simulink model "rate_control_integrado_controlePD_r2018b"  (R2018b)
settings: Solver=FixedStepAuto  StartTime=0.0  StopTime=tsim  FixedStep=1/100  RelTol=1e-3
values from neighbouring files (symbols this model uses):
  Beff = 50    [Ex5.m]
  Jeff = 2.2    [Ex5.m]
  K = 17.7    [Ex5.m]
  Kd = (2*qsi*wn*Jeff - Beff)/K    (= -0.338983050847)    [Ex5.m]
  Kp = (wn^2*Jeff)/K    (= 12.4293785311)    [Ex5.m]
  L = [0.5;0.5;0.5]    [Ex5.m]
  N = 10    [Ex5.m]
  r = 1    [Ex5.m]
  SP_theta = ThetaA0    [Ex5.m]
  ThetaA0 = [10;20;30]    [Ex5.m]
  W_0 = [1 2 3]'    [Ex5.m]
  XdotC0 = [.2 -.3 -.2]'    [Ex5.m]
settings Model: Creator=Karoline  LastModifiedBy=Karoline
settings DataIOCC: ExternalInput=[L, ThetaA]
settings SFSimCC: SimUseLocalCustomCode=off
settings RTWCC: RTWUseLocalCustomCode=off
settings CodeAppCC: StateflowObjectComments=on

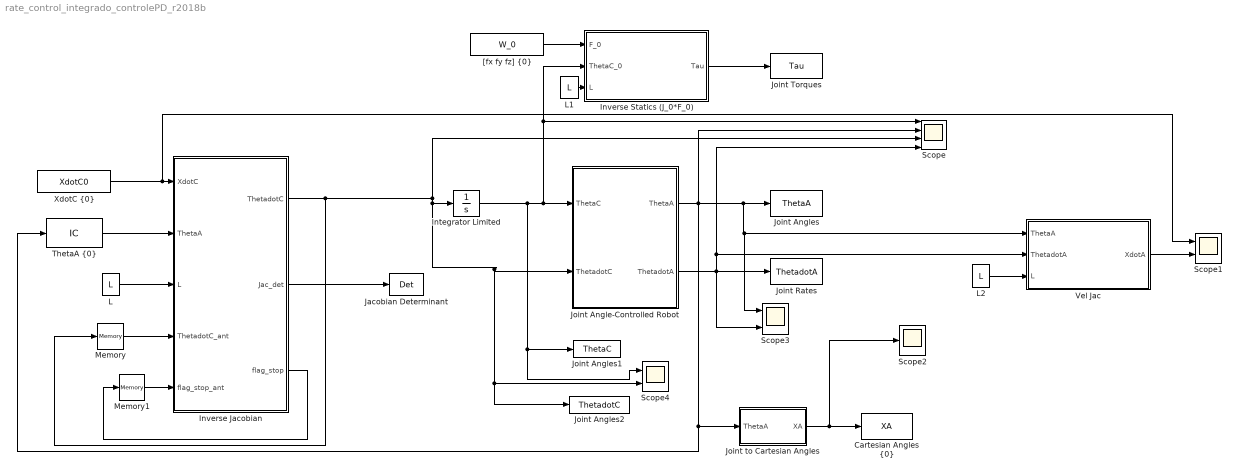
== system rate_control_integrado_controlePD_r2018b ==
  "Cartesian Angles {0}" : ToWorkspace  VariableName=XA  SampleTime=-1
      settings: Save2DSignal=2-D array (concatenate along first dimension)
  Integrator Limited : Integrator  InitialCondition=ThetaA0  LimitOutput=on  UpperSaturationLimit=[170, 170, 170]  LowerSaturationLimit=[-170, -170, -170]
  Inverse Jacobian : MATLAB Function  TreatAsAtomicUnit=on
  Inverse Statics (J_0*F_0) : MATLAB Function  TreatAsAtomicUnit=on
  Jacobian Determinant : ToWorkspace  VariableName=Det  SampleTime=-1
  Joint Angle-Controlled Robot : Subsystem
  Joint Angles : ToWorkspace  VariableName=ThetaA  SampleTime=-1
  Joint Angles1 : ToWorkspace  VariableName=ThetaC  SampleTime=-1
  Joint Angles2 : ToWorkspace  VariableName=ThetadotC  SampleTime=-1
  Joint Rates : ToWorkspace  VariableName=ThetadotA  SampleTime=-1
  Joint Torques : ToWorkspace  VariableName=Tau  SampleTime=-1
  Joint to Cartesian Angles : Subsystem
  L : Constant  Value=L
  L1 : Constant  Value=L
  L2 : Constant  Value=L
  Memory : Memory  InitialCondition=[0; 0; 0]
  Memory1 : Memory
  Scope : Scope  NumInputPorts=4
  Scope1 : Scope  NumInputPorts=2
  Scope2 : Scope
  Scope3 : Scope  NumInputPorts=2
  Scope4 : Scope  NumInputPorts=2
  "ThetaA {0}" : InitialCondition  Value=ThetaA0
  Vel Jac : MATLAB Function  TreatAsAtomicUnit=on
  "XdotC {0}" : Constant  Value=XdotC0
  "[fx fy fz] {0}" : Constant  Value=W_0
  wires:
  Inverse Jacobian/1(ThetadotC) -> Memory/1, Joint Angles2/1, Scope4/2, Joint Angle-Controlled Robot/2(ThetadotC), Integrator Limited/1, Scope/3
  Inverse Jacobian/2(Jac_det) -> Jacobian Determinant/1
  Integrator Limited/1 -> Joint Angles1/1, Scope4/1, Scope/1, Inverse Statics (J_0*F_0)/2(ThetaC_0), Joint Angle-Controlled Robot/1(ThetaC)
  Joint Angle-Controlled Robot/1(ThetaA) -> Scope/2, Scope3/1, Vel Jac/1(ThetaA), Joint Angles/1, "ThetaA {0}"/1, Joint to Cartesian Angles/1(ThetaA)
  Joint Angle-Controlled Robot/2(ThetadotA) -> Scope3/2, Scope/4, Vel Jac/2(ThetadotA), Joint Rates/1
  Inverse Statics (J_0*F_0)/1(Tau) -> Joint Torques/1
  Joint to Cartesian Angles/1(XA) -> Scope2/1, "Cartesian Angles {0}"/1
  "[fx fy fz] {0}"/1 -> Inverse Statics (J_0*F_0)/1(F_0)
  "ThetaA {0}"/1 -> Inverse Jacobian/2(ThetaA)
  L/1 -> Inverse Jacobian/3(L)
  L1/1 -> Inverse Statics (J_0*F_0)/3(L)
  L2/1 -> Vel Jac/3(L)
  Vel Jac/1(XdotA) -> Scope1/2
  Inverse Jacobian/3(flag_stop) -> Memory1/1
  "XdotC {0}"/1 -> Scope1/1, Inverse Jacobian/1(XdotC)
  Memory/1 -> Inverse Jacobian/4(ThetadotC_ant)
  Memory1/1 -> Inverse Jacobian/5(flag_stop_ant)

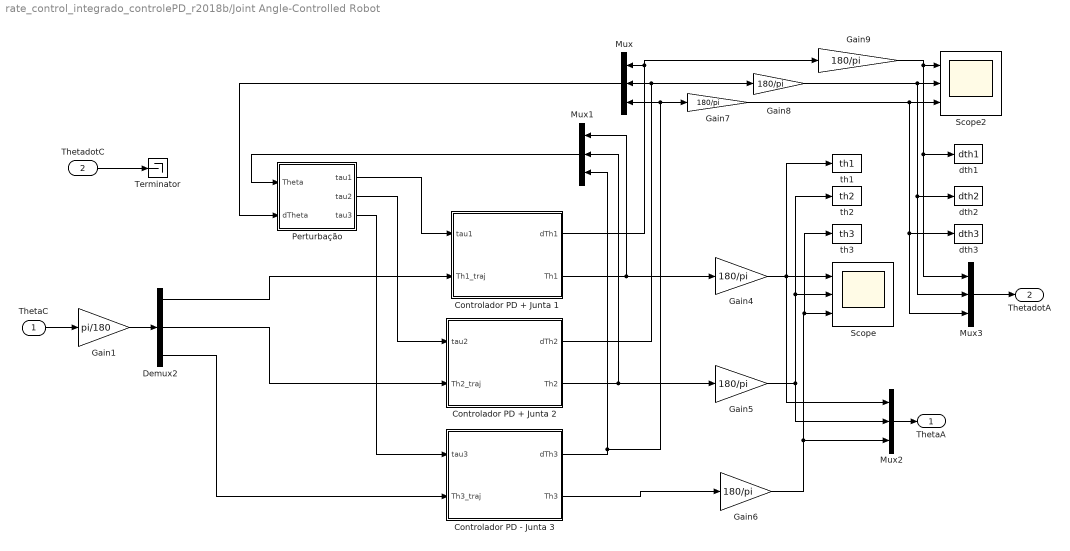
== system rate_control_integrado_controlePD_r2018b/Joint Angle-Controlled Robot ==
  ThetaC : Inport
  ThetadotC : Inport  Port=2
  Controlador PD + Junta 1 : Subsystem
  Controlador PD + Junta 2 : Subsystem
  Controlador PD - Junta 3 : Subsystem
  Demux2 : Demux  Outputs=3
  Gain1 : Gain  Gain=pi/180
  Gain{4..9} (6 alike) : Gain  Gain=180/pi
  Mux{,1..3} (4 alike) : Mux  Inputs=3
  Perturbação : Subsystem
  Scope : Scope  NumInputPorts=3
  Scope2 : Scope  NumInputPorts=3
  Terminator : Terminator
  dth1 : ToWorkspace  VariableName=dth1  SampleTime=-1
  dth2 : ToWorkspace  VariableName=dth2  SampleTime=-1
  dth3 : ToWorkspace  VariableName=dth3  SampleTime=-1
  th1 : ToWorkspace  VariableName=th1  SampleTime=-1
  th2 : ToWorkspace  VariableName=th2  SampleTime=-1
  th3 : ToWorkspace  VariableName=th3  SampleTime=-1
  ThetaA : Outport
  ThetadotA : Outport  Port=2
  wires:
  Gain8/1 -> Mux3/2, dth2/1, Scope2/2
  Gain9/1 -> Mux3/1, dth1/1, Scope2/1
  Controlador PD - Junta 3/1("dTh3 ") -> Mux1/3, Mux/3, Gain7/1
  Perturbação/3(tau3) -> Controlador PD - Junta 3/1(tau3)
  Gain7/1 -> Mux3/3, dth3/1, Scope2/3
  Gain5/1 -> th2/1, Scope/2, Mux2/2
  Controlador PD - Junta 3/2(Th3) -> Gain6/1
  Controlador PD + Junta 2/1("dTh2 ") -> Mux/2, Gain8/1
  Mux/1 -> Perturbação/2(dTheta)
  Controlador PD + Junta 2/2(Th2) -> Mux1/2, Gain5/1
  Gain4/1 -> th1/1, Mux2/1, Scope/1
  Controlador PD + Junta 1/1("dTh1 ") -> Mux/1, Gain9/1
  Perturbação/2(tau2) -> Controlador PD + Junta 2/1(tau2)
  Gain6/1 -> Mux2/3, th3/1, Scope/3
  Controlador PD + Junta 1/2(Th1) -> Mux1/1, Gain4/1
  Perturbação/1(tau1) -> Controlador PD + Junta 1/1(tau1)
  Mux1/1 -> Perturbação/1(Theta)
  ThetaC/1 -> Gain1/1
  Demux2/1 -> Controlador PD + Junta 1/2(Th1_traj)
  Demux2/2 -> Controlador PD + Junta 2/2(Th2_traj)
  Demux2/3 -> Controlador PD - Junta 3/2(Th3_traj)
  Mux2/1 -> ThetaA/1
  Mux3/1 -> ThetadotA/1
  Gain1/1 -> Demux2/1
  ThetadotC/1 -> Terminator/1

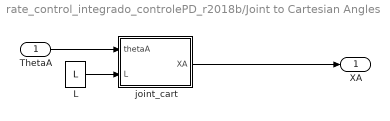
== system rate_control_integrado_controlePD_r2018b/Joint to Cartesian Angles ==
  ThetaA : Inport
  L : Constant  Value=L
  joint_cart : MATLAB Function  TreatAsAtomicUnit=on
  XA : Outport
  wires:
  ThetaA/1 -> joint_cart/1(thetaA)
  joint_cart/1(XA) -> XA/1
  L/1 -> joint_cart/2(L)

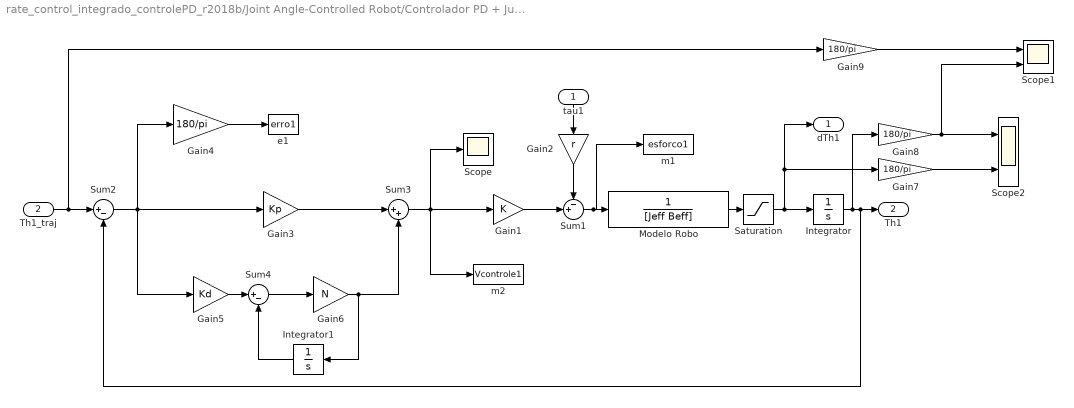
== system rate_control_integrado_controlePD_r2018b/Joint Angle-Controlled Robot/Controlador PD + Junta 1 ==
  tau1 : Inport
  Th1_traj : Inport  Port=2
  Gain1 : Gain  Gain=K
  Gain2 : Gain  Gain=r
  Gain3 : Gain  Gain=Kp
  Gain{4,7..9} (4 alike) : Gain  Gain=180/pi
  Gain5 : Gain  Gain=Kd
  Gain6 : Gain  Gain=N
  Integrator : Integrator  InitialCondition=SP_theta(1)*pi/180
  Integrator1 : Integrator
  Modelo Robo : TransferFcn  Denominator=[Jeff Beff]
  Saturation : Saturate  UpperLimit=10*pi/180  LowerLimit=-10*pi/180
  Scope : Scope
  Scope1 : Scope  NumInputPorts=2
  Scope2 : Scope  NumInputPorts=2
  Sum1 : Sum  Inputs=-+|
  Sum2 : Sum  Inputs=|+-
  Sum3 : Sum  Inputs=|++
  Sum4 : Sum  Inputs=|+-
  e1 : ToWorkspace  VariableName=erro1  SampleTime=-1
  m1 : ToWorkspace  VariableName=esforco1  SampleTime=-1
  m2 : ToWorkspace  VariableName=Vcontrole1  SampleTime=-1
  "dTh1 " : Outport
  Th1 : Outport  Port=2
  wires:
  tau1/1 -> Gain2/1
  Gain1/1 -> Sum1/2
  Sum1/1 -> m1/1, Modelo Robo/1
  Integrator/1 -> Gain8/1, Th1/1, Sum2/2
  Th1_traj/1 -> Gain9/1, Sum2/1
  Gain2/1 -> Sum1/1
  Sum2/1 -> Gain5/1, Gain3/1, Gain4/1
  Gain4/1 -> e1/1
  Gain3/1 -> Sum3/1
  Gain5/1 -> Sum4/1
  Sum4/1 -> Gain6/1
  Gain6/1 -> Sum3/2, Integrator1/1
  Integrator1/1 -> Sum4/2
  Sum3/1 -> m2/1, Scope/1, Gain1/1
  Modelo Robo/1 -> Saturation/1
  Saturation/1 -> "dTh1 "/1, Gain7/1, Integrator/1
  Gain8/1 -> Scope1/2, Scope2/1
  Gain7/1 -> Scope2/2
  Gain9/1 -> Scope1/1

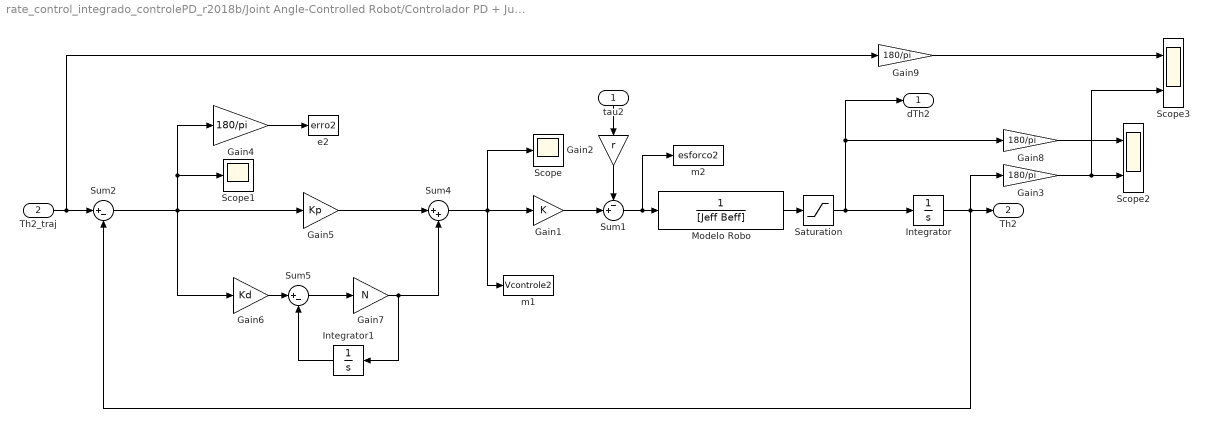
== system rate_control_integrado_controlePD_r2018b/Joint Angle-Controlled Robot/Controlador PD + Junta 2 ==
  tau2 : Inport
  Th2_traj : Inport  Port=2
  Gain1 : Gain  Gain=K
  Gain2 : Gain  Gain=r
  Gain{3..4,8..9} (4 alike) : Gain  Gain=180/pi
  Gain5 : Gain  Gain=Kp
  Gain6 : Gain  Gain=Kd
  Gain7 : Gain  Gain=N
  Integrator : Integrator  InitialCondition=SP_theta(2)*pi/180
  Integrator1 : Integrator
  "Modelo Robo " : TransferFcn  Denominator=[Jeff Beff]
  Saturation : Saturate  UpperLimit=10*pi/180  LowerLimit=-10*pi/180
  Scope : Scope
  Scope1 : Scope
  Scope2 : Scope  NumInputPorts=2
  Scope3 : Scope  NumInputPorts=2
  Sum1 : Sum  Inputs=-+|
  Sum2 : Sum  Inputs=|+-
  Sum4 : Sum  Inputs=|++
  Sum5 : Sum  Inputs=|+-
  e2 : ToWorkspace  VariableName=erro2  SampleTime=-1
  m1 : ToWorkspace  VariableName=Vcontrole2  SampleTime=-1
  m2 : ToWorkspace  VariableName=esforco2  SampleTime=-1
  "dTh2 " : Outport
  Th2 : Outport  Port=2
  wires:
  tau2/1 -> Gain2/1
  Gain1/1 -> Sum1/2
  Sum1/1 -> m2/1, "Modelo Robo "/1
  Integrator/1 -> Gain3/1, Th2/1, Sum2/2
  Gain2/1 -> Sum1/1
  Gain4/1 -> e2/1
  Gain5/1 -> Sum4/1
  Sum2/1 -> Gain4/1, Scope1/1, Gain6/1, Gain5/1
  Integrator1/1 -> Sum5/2
  Sum5/1 -> Gain7/1
  Gain6/1 -> Sum5/1
  Gain7/1 -> Sum4/2, Integrator1/1
  Sum4/1 -> m1/1, Scope/1, Gain1/1
  "Modelo Robo "/1 -> Saturation/1
  Saturation/1 -> Gain8/1, "dTh2 "/1, Integrator/1
  Gain3/1 -> Scope3/2, Scope2/2
  Gain8/1 -> Scope2/1
  Th2_traj/1 -> Gain9/1, Sum2/1
  Gain9/1 -> Scope3/1

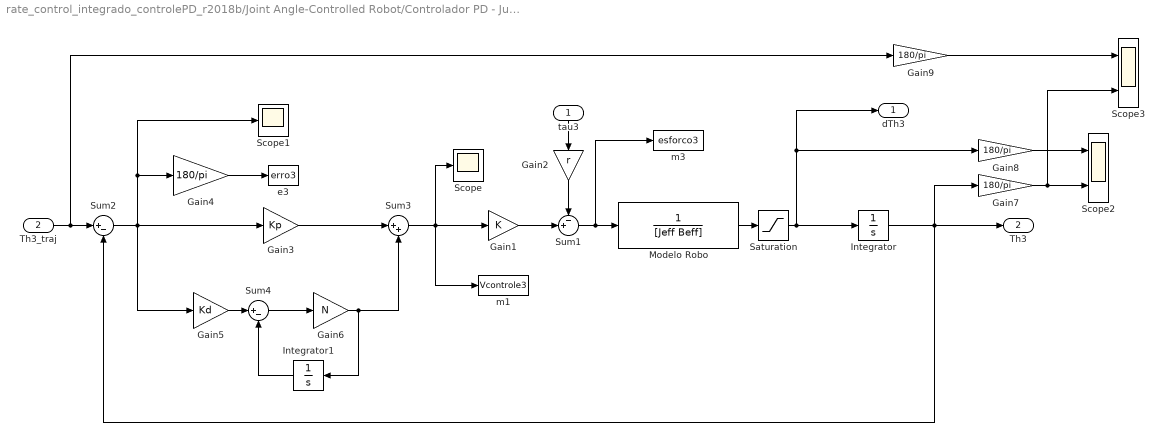
== system rate_control_integrado_controlePD_r2018b/Joint Angle-Controlled Robot/Controlador PD - Junta 3 ==
  tau3 : Inport
  Th3_traj : Inport  Port=2
  Gain1 : Gain  Gain=K
  Gain2 : Gain  Gain=r
  Gain3 : Gain  Gain=Kp
  Gain{4,7..9} (4 alike) : Gain  Gain=180/pi
  Gain5 : Gain  Gain=Kd
  Gain6 : Gain  Gain=N
  Integrator : Integrator  InitialCondition=SP_theta(3)*pi/180
  Integrator1 : Integrator
  Modelo Robo : TransferFcn  Denominator=[Jeff Beff]
  Saturation : Saturate  UpperLimit=10*pi/180  LowerLimit=-10*pi/180
  Scope : Scope
  Scope1 : Scope
  Scope2 : Scope  NumInputPorts=2
  Scope3 : Scope  NumInputPorts=2
  Sum1 : Sum  Inputs=-+|
  Sum2 : Sum  Inputs=|+-
  Sum3 : Sum  Inputs=|++
  Sum4 : Sum  Inputs=|+-
  e3 : ToWorkspace  VariableName=erro3  SampleTime=-1
  m1 : ToWorkspace  VariableName=Vcontrole3  SampleTime=-1
  m3 : ToWorkspace  VariableName=esforco3  SampleTime=-1
  "dTh3 " : Outport
  Th3 : Outport  Port=2
  wires:
  tau3/1 -> Gain2/1
  Gain1/1 -> Sum1/2
  Sum1/1 -> m3/1, Modelo Robo/1
  Integrator/1 -> Sum2/2, Gain7/1, Th3/1
  Th3_traj/1 -> Gain9/1, Sum2/1
  Gain2/1 -> Sum1/1
  Gain4/1 -> e3/1
  Gain3/1 -> Sum3/1
  Sum2/1 -> Gain4/1, Scope1/1, Gain5/1, Gain3/1
  Integrator1/1 -> Sum4/2
  Sum4/1 -> Gain6/1
  Gain5/1 -> Sum4/1
  Gain6/1 -> Sum3/2, Integrator1/1
  Sum3/1 -> m1/1, Scope/1, Gain1/1
  Modelo Robo/1 -> Saturation/1
  Saturation/1 -> Gain8/1, "dTh3 "/1, Integrator/1
  Gain7/1 -> Scope2/2, Scope3/2
  Gain8/1 -> Scope2/1
  Gain9/1 -> Scope3/1

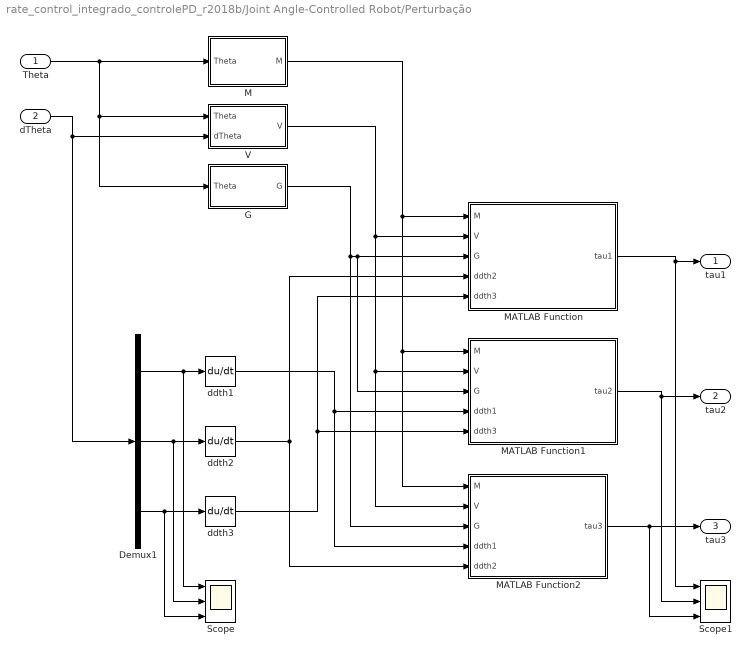
== system rate_control_integrado_controlePD_r2018b/Joint Angle-Controlled Robot/Perturbação ==
  Theta : Inport
  dTheta : Inport  Port=2
  Demux1 : Demux  Outputs=3
  G : Subsystem
  M : Subsystem
  MATLAB Function : MATLAB Function  TreatAsAtomicUnit=on
  MATLAB Function1 : MATLAB Function  TreatAsAtomicUnit=on
  MATLAB Function2 : MATLAB Function  TreatAsAtomicUnit=on
  Scope : Scope  NumInputPorts=3
  Scope1 : Scope  NumInputPorts=3
  V : Subsystem
  ddth1 : Derivative
  ddth2 : Derivative
  ddth3 : Derivative
  tau1 : Outport
  tau2 : Outport  Port=2
  tau3 : Outport  Port=3
  wires:
  dTheta/1 -> Demux1/1, V/2(dTheta)
  G/1(G) -> MATLAB Function2/3(G), MATLAB Function1/3(G), MATLAB Function/3(G)
  V/1(V) -> MATLAB Function/2(V), MATLAB Function1/2(V), MATLAB Function2/2(V)
  M/1(M) -> MATLAB Function2/1(M), MATLAB Function1/1(M), MATLAB Function/1(M)
  Theta/1 -> M/1(Theta), G/1(Theta), V/1(Theta)
  Demux1/1 -> Scope/1, ddth1/1
  Demux1/2 -> Scope/2, ddth2/1
  Demux1/3 -> Scope/3, ddth3/1
  ddth1/1 -> MATLAB Function2/4(ddth1), MATLAB Function1/4(ddth1)
  ddth3/1 -> MATLAB Function/5(ddth3), MATLAB Function1/5(ddth3)
  ddth2/1 -> MATLAB Function/4(ddth2), MATLAB Function2/5(ddth2)
  MATLAB Function/1(tau1) -> Scope1/1, tau1/1
  MATLAB Function1/1(tau2) -> tau2/1, Scope1/2
  MATLAB Function2/1(tau3) -> tau3/1, Scope1/3

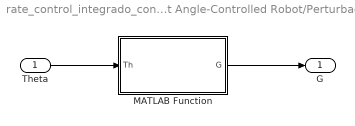
== system rate_control_integrado_controlePD_r2018b/Joint Angle-Controlled Robot/Perturbação/G ==
  Theta : Inport
  MATLAB Function : MATLAB Function  TreatAsAtomicUnit=on
  G : Outport
  wires:
  Theta/1 -> MATLAB Function/1(Th)
  MATLAB Function/1(G) -> G/1

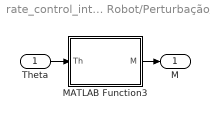
== system rate_control_integrado_controlePD_r2018b/Joint Angle-Controlled Robot/Perturbação/M ==
  Theta : Inport
  MATLAB Function3 : MATLAB Function  TreatAsAtomicUnit=on
  M : Outport
  wires:
  Theta/1 -> MATLAB Function3/1(Th)
  MATLAB Function3/1(M) -> M/1

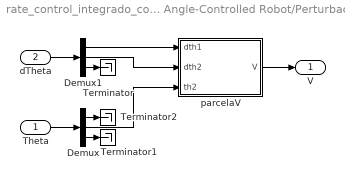
== system rate_control_integrado_controlePD_r2018b/Joint Angle-Controlled Robot/Perturbação/V ==
  Theta : Inport
  dTheta : Inport  Port=2
  Demux : Demux  Outputs=3
  Demux1 : Demux  Outputs=3
  Terminator : Terminator
  Terminator1 : Terminator
  Terminator2 : Terminator
  parcelaV : MATLAB Function  TreatAsAtomicUnit=on
  V : Outport
  wires:
  Theta/1 -> Demux/1
  dTheta/1 -> Demux1/1
  Demux1/1 -> parcelaV/1(dth1)
  Demux1/2 -> parcelaV/2(dth2)
  Demux/2 -> parcelaV/3(th2)
  parcelaV/1(V) -> V/1
  Demux1/3 -> Terminator/1
  Demux/1 -> Terminator2/1
  Demux/3 -> Terminator1/1

== matlab function rate_control_integrado_controlePD_r2018b/Inverse Jacobian ==
  data: XdotC input; ThetadotC output; ThetaA input; Jac_det output; L input; flag_stop output; ThetadotC_ant input; flag_stop_ant input
function [ThetadotC,Jac_det,flag_stop] = invjac(XdotC,ThetaA,L,ThetadotC_ant, flag_stop_ant)

vel_lim = 10; % º/seg

if (abs(ThetadotC_ant(1))>=vel_lim || abs(ThetadotC_ant(2))>=vel_lim || abs(ThetadotC_ant(3))>=vel_lim) || flag_stop_ant == 1
    ThetadotC = [0; 0; 0];
    flag_stop = 1;
    Jac_det = 0; %Jac_det_ant;
else
    [J] = jacobianRRR(ThetaA,L);
    Jac_det = det(J);
%     Jinv = inv(J);
    ThetadotC = J\XdotC;  
    
    flag_stop = 0;
end


end

== matlab function rate_control_integrado_controlePD_r2018b/Inverse Statics (J_0*F_0) ==
  data: F_0 input; Tau output; ThetaC_0 input; L input
function Tau = jacob_calcul(F_0,ThetaC_0,L)


J_0 = jacobianRRR(ThetaC_0,L); % jacobiano

Tau = J_0'*F_0;

== matlab function rate_control_integrado_controlePD_r2018b/Joint to Cartesian Angles/joint_cart ==
  data: thetaA input; XA output; L input
function XA = joint_cart(thetaA,L)


srelb_user = [0;0;0];
srelb = utoi(srelb_user);

trelw_user = [L(3);0;0];
trelw = utoi(trelw_user);

[trels]=where_robot(thetaA,trelw,srelb,L);

XA = itou(trels);

== matlab function rate_control_integrado_controlePD_r2018b/Vel Jac ==
  data: ThetaA input; ThetadotA input; L input; XdotA output
function XdotA = jac(ThetaA,ThetadotA,L)


J_0 = jacobianRRR(ThetaA,L); % jacobiano

XdotA = J_0*ThetadotA;

== matlab function rate_control_integrado_controlePD_r2018b/Joint Angle-Controlled Robot/Perturbação/G/MATLAB Function ==
  data: Th input; G output
function G = calcul_G(Th)

th1 = Th(1);
th2 = Th(2);
th3 = Th(3);

G = [(1617*cos(th1 + th2))/100 + (3871*cos(th1))/100;...
    (1617*cos(th1 + th2))/100;...
    0];

== matlab function rate_control_integrado_controlePD_r2018b/Joint Angle-Controlled Robot/Perturbação/M/MATLAB Function3 ==
  data: Th input; M output
function M = calcul_M(Th)

th1 = Th(1);
th2 = Th(2);
th3 = Th(3);

M = [(33*cos(th2))/20 + 29/10, (33*cos(th2))/40 + 37/40, 1/10;...
     (33*cos(th2))/40 + 37/40,                    37/40, 1/10;...
                         1/10,                     1/10, 1/10];

== matlab function rate_control_integrado_controlePD_r2018b/Joint Angle-Controlled Robot/Perturbação/MATLAB Function ==
  data: M input; V input; tau1 output; G input; ddth2 input; ddth3 input
function tau1  = calcul_dk1(M,V,G,ddth2,ddth3)


% tau1 = m12*ddth2 + m13*ddth3 + v1 + g1;
tau1 = M(1,2)*ddth2 + M(1,3)*ddth3 + V(1,1) + G(1);

== matlab function rate_control_integrado_controlePD_r2018b/Joint Angle-Controlled Robot/Perturbação/MATLAB Function1 ==
  data: M input; V input; tau2 output; G input; ddth1 input; ddth3 input
function tau2  = calcul_dk2(M,V,G,ddth1, ddth3)


% tau2 = m21*ddth1 + m23*ddth3 + v2 + g2;
tau2 = M(2,1)*ddth1 + M(2,3)*ddth3 + V(2,1) + G(2);

== matlab function rate_control_integrado_controlePD_r2018b/Joint Angle-Controlled Robot/Perturbação/MATLAB Function2 ==
  data: M input; V input; tau3 output; G input; ddth1 input; ddth2 input
function tau3  = calcul_dk3(M, V, G, ddth1, ddth2)



% tau3 = m31*ddth1 + m32*ddth2 + v3 + g3;
tau3 = M(3,1)*ddth1 + M(3,2)*ddth2 + V(3,1) + G(3);

== matlab function rate_control_integrado_controlePD_r2018b/Joint Angle-Controlled Robot/Perturbação/V/parcelaV ==
  data: dth1 input; V output; dth2 input; th2 input
function V = parcelaV(dth1,dth2,th2)
%#codegen

%    This function was generated by the Symbolic Math Toolbox version 8.2.
%    18-Oct-2019 15:37:48

t2 = sin(th2);
V = [dth2.^2.*t2.*(-3.3e1./4.0e1)-dth1.*dth2.*t2.*(3.3e1./2.0e1);dth1.^2.*t2.*(3.3e1./4.0e1);0.0];
